simulink model "ex6_4"  (R2018a)
settings: Solver=VariableStepAuto  StartTime=0.0  StopTime=60  RelTol=1e-5
settings Model: Creator=HUAWEI  LastModifiedBy=HUAWEI

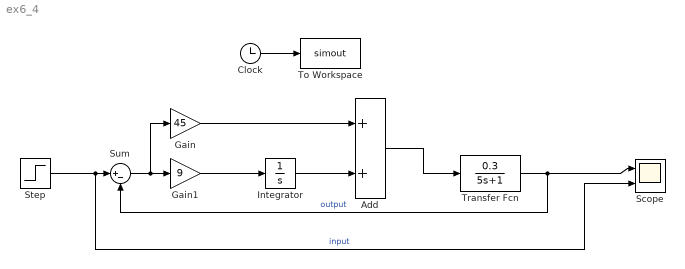
== system ex6_4 ==
  Add : Sum  Inputs=2
  Clock : Clock
  Gain : Gain  Gain=45
  Gain1 : Gain  Gain=9
  Integrator : Integrator
  Scope : Scope  NumInputPorts=2
  Step : Step  SampleTime=0
  Sum : Sum  Inputs=|+-
  To Workspace : ToWorkspace  VariableName=simout  SaveFormat=Timeseries  SampleTime=-1
  Transfer Fcn : TransferFcn  Numerator=[0.3]  Denominator=[5 1]
  wires:
  Step/1 -> Scope/2, Sum/1  "input"
  Clock/1 -> To Workspace/1
  Add/1 -> Transfer Fcn/1
  Transfer Fcn/1 -> Sum/2, Scope/1  "output"
  Gain/1 -> Add/1
  Integrator/1 -> Add/2
  Gain1/1 -> Integrator/1
  Sum/1 -> Gain1/1, Gain/1
